simulink library "ITKLib"  (R2022b)
settings: Solver=FixedStepDiscrete  StartTime=0.0  StopTime=10.0  FixedStep=0.01  RelTol=1e-3  EnableMultiTasking=on
values from neighbouring files (symbols this model uses):
  Glb_WhlRollgRd_SC = single(0.36)    [init_Global.m]
undefined symbols (not defined in the file or in its folder): docblock, SlDemoSign, SlDemoSign_Positive_SC, TaskTime_100ms_SC, TaskTime_10ms_SC, VehRefSpd_vMaxRefSpd_C
libraries: simulink x51, $bdroot x45, ITKLib_V14 x1
(part 3 of 10)

== system ITKLib/TimeCounter ==
  Accum : Subsystem  RTWFcnName=Accum  RTWFileName=MCC_Mdl_Lib  mask(Accum){}
      mask help:
      | The main purpose of the Accum module is to achieve the accumulation of single floating-point data. Usually, when a large floating-point data is added to a small floating-point data, the data precision will be lost and the accumulation will not be possible. At this time, the small floating-point data can be accumulated separately into a large floating-point data (IncLim), and then added with another large floating-point data;
      | Input signals:
      | In : single data type, small floating-point data, for example 0.01 0.001 0.0001;
      | IncLim: single data type, the upper limiter of increasing step, for example 0.1 1 10;
      | Rst: single data type, reset flag, when Rst is true, the out is 0;
      | IV: single data type, intial value;
      | Output signals:
      | Out: single data type;
      |
      | For example, In = 0.01, IncLim = 1,
      | if without this module, when the maximum accumulation value is 100000;
      | if with this module, the maximum accumulation value is 9999999999;
      |
      | Simulink Custom Model Library, created by MCC and YZK.
      settings: MinAlgLoopOccurrences=on  RTWFcnNameOpts=User specified  RTWFileNameOpts=User specified
      mask Display:
      | color('red')
      | % plot(0.15+0.05*[0 1 1 3 3 5 5 7 7 9 9 11 11 13 13 15 15 16],0.15+0.1*[0 0 2 2 4 4 0 0 2 2 4 4 6 6 8 8 0 0] )
      | % color('blue')
      | % text(0.25,0.15,'IV')
      | color('green');
      | image('AccumImage.jpg', [0.15, 0.1, 0.75, 0.8]);
      | text(1,0,'ITK','horizontalAlignment','right','verticalAlignment','bottom');
  CountR : Subsystem  RTWFcnName=CountR  RTWFileName=BoschITK_Mdl_Lib  mask(CountR){MAX=uint16(400)}
      mask prompts: MAX "Maximum value of counter"
      mask help:
      | Increments and outputs the counter every calling (step) by value 1 when enabled and set saturation flag to TRUE when counter reaches limit.
      |
      | Reset by external request.
      |
      | Simulink Custom Model Library, created by MCC.
      settings: RTWFcnNameOpts=User specified  RTWFileNameOpts=User specified
      settings: AttributesFormatString=|
      | CountR
      | Cnt_Max=%<MAX>
      mask Display:
      | color('red')
      | plot(0.15+0.05*[0 1 1 2 2 3 3 4 4 5 5 6 6 7 7 8 8 9 9 10 10 11 11 12 12 13 13 14],0.15+0.1*[0 0 1 1 2 2 3 3 4 4 0 0 1 1 2 2 3 3 4 4 5 5 6 6 7 7 0 0] )
      | color('green');
      | text(1,0,'ITK','horizontalAlignment','right','verticalAlignment','bottom');
  CountRIV : Subsystem  RTWFcnName=CountR_IV  RTWFileName=BoschITK_Mdl_Lib  mask(CountRIV){MAX=uint16(400)}
      mask prompts: MAX "Maximum value of counter"
      mask help:
      | Increments and outputs the counter by value 1 which starts from an initial value every calling (step) when enabled and set saturation flag to TRUE when counter reaches limit.
      |
      | Reset by external request.
      |
      | Simulink Custom Model Library, created by MCC.
      settings: RTWFcnNameOpts=User specified  RTWFileNameOpts=User specified
      settings: AttributesFormatString=|
      | CountRIV
      | Cnt_Max=%<MAX>
      mask Display:
      | color('red')
      | plot(0.15+0.05*[0 1 1 2 2 3 3 4 4 5 5 6 6 7 7 8 8 9 9 10 10 11 11 12 12 13 13 14],0.15+0.1*[0 0 1 1 2 2 3 3 4 4 0 0 1 1 2 2 3 3 4 4 5 5 6 6 7 7 0 0] )
      | color('blue')
      | text(0.25,0.15,'IV')
      | color('green');
      | text(1,0,'ITK','horizontalAlignment','right','verticalAlignment','bottom');
  CounterRStep : Subsystem  RTWFcnName=CounterR_Step  RTWFileName=BoschITK_Mdl_Lib  mask(CounterRStep){Cnt_Max=uint16(400)}
      mask prompts: Cnt_Max "Maximum value of counter"
      mask help:
      | Increments and outputs the counter every calling (step) by value "Inc" when enabled and set saturation flag to TRUE when counter reaches limit.
      |
      | Reset by external request.
      |
      | Simulink Custom Model Library, created by MCC.
      mask init:
      | if Cnt_Max > 65535;
      |     helpdlg('Cnt_Max cannot be greater than 4294967295 !','ERROR1');
      | end
      | Cnt_Max = min(Cnt_Max,65535);
      settings: RTWFcnNameOpts=User specified  RTWFileNameOpts=User specified
      settings: AttributesFormatString=|
      | CounterRStep
      | Cnt_Max=%<Cnt_Max>
      mask Display:
      | color('red')
      | plot(0,0,100,100,[12,10,8,10,10],[87,90,87,90,10],[88,90,88,90,10],[7,10,12,10,10],[90,80,80,70,70,60,60,50,50,40,40,30,30,20,20],[80,80,70,70,60,60,50,50,40,40,30,30,20,20,10])
      | color('green');
      | text(100,0,'ITK','horizontalAlignment','right','verticalAlignment','bottom');
  DebCnt : Subsystem  RTWFcnName=Debounce_OBD  RTWFileName=JaevRI_Mdl_Lib  mask(DebCnt){}
      mask help:
      | Inputs:
      |              bErr: Error signal(s)  (i.e. vector of continuous test runs), boolean signal;
      |              FailThd: counter a value (for each bErr signal), int16 signal;
      |              RcvThd: counter a value (for each bErr signal), int16 signal;
      |              IncFail: increment Fault counter, >0, int16 signal;
      |              DecRcv: decrement Recovery counter, <0, int16 signal;
      |              bEna: bErr is 0 when bEna=0, detecting whether bErr is 1 when bEna=1, boolean signal;
      |              bRst: reset flag of bErr(bErr is 0 when bRst=1), boolean signal;
      | Outputs :
      |                 bFaild: testFaild  (Bit 0)
      | So Counters are in numbers of timer ticks of TaskTime( for example, 0.01s);
      | E.g. if FailThd is 20, RecThd is -4, Increment counter is 5 and decrement counter -3 when bEna is 1and bRst is 0, the initial counter is 0,
      | then fail times are: 20*0.01/5 = 0.04 sec, recovery times are: (-4-20)*0.01/(-3) = 0.08 sec;
      |
      | Simulink Custom Model Library, created by MCC.
      settings: RTWFcnNameOpts=User specified  RTWFileNameOpts=User specified
      mask Display:
      | % color('black');
      | % plot([0.2,0.2],[0.1,0.9]);
      | % plot([0.205,0.205],[0.1,0.9]);
      | % plot([0.2,0.8],[0.8,0.8]);
      | % plot([0.2,0.8],[0.65,0.65]);
      | % plot([0.2,0.8],[0.45,0.45]);
      | % plot([0.2,0.8],[0.25,0.25]);
      | % plot([0.2,0.8],[0.1,0.1]);
      | port_label('input',1,'bErr');
      | port_label('input',2,'bRst');
      | port_label('input',3,'bEna');
      | port_label('input',4,'FailThd');
      | port_label('input',5,'RcvThd');
      | port_label('input',6,'IncFail');
      | port_label('input',7,'DecRcv');
      | port_label('output',1,'bFaild');
      | % color('cyan');
      | % plot([0.3,0.3],[0.1,0.9]);
      | % plot([0.4,0.4],[0.1,0.9]);
      | % plot([0.5,0.5],[0.1,0.9]);
      | % plot([0.6,0.6],[0.1,0.9]);
      | % plot([0.7,0.7],[0.1,0.9]);
      | % plot([0.8,0.8],[0.1,0.9]);
      | % color('orange');
      | % plot([0.2,0.3,0.3,0.6,0.6,0.8],[0.85,0.85,0.8,0.8,0.85,0.85]);
      | % plot([0.2,0.5,0.5,0.6,0.6,0.8],[0.7,0.7,0.65,0.65,0.7,0.7]);
      | % color('blue');
      | % plot([0.2,0.3,0.4,0.5,0.5,0.6,0.7,0.8],[0.45,0.55,0.35,0.35,0.45,0.45,0.6,0.6]);
      | % color('red');
      | % plot([0.2,0.7,0.7,0.8],[0.25,0.25,0.3,0.3]);
      | % color('green');
      | % plot([0.2,0.4,0.4,0.5,0.5,0.8],[0.1,0.1,0.15,0.15,0.1,0.1]);
      | color('green');
      | text(1,0,'ITK','horizontalAlignment','right','verticalAlignment','bottom');
  Debounce : Subsystem  RTWFcnName=Debounce  RTWFileName=BoschITK_Mdl_Lib  mask(Debounce){IV=0}
      mask prompts: IV "Initial output value"
      mask help:
      | This block enables debounce action of input signal "In" :
      | - if it changes from fasle to true, "Out" will be set to true after TAct time
      | - if it changes from true to false, "Out" will be set to fasle after TDeact temps
      | - The initial value is given via the parameter window
      |
      | Besides,
      | "In" -- boolean type
      | R -- Reset flag，boolean type
      | TAct -- time in s, single type
      | TDeact -- time in s, single type
      | dT -- Sample time in s, single type
      |
      | Simulink Custom Model Library, created by MCC.
      mask init:
      | %val = get_param(gcb, 'IV');
      | %set_param([gcb, '/RS Latch'], 'IV', num2str(val))
      settings: RTWFcnNameOpts=User specified  RTWFileNameOpts=User specified
      settings: AttributesFormatString=|
      | Debounce
      | Init = %<IV>
      mask Display:
      | color('red')
      | plot([0.10 0.20 0.20],[0.55 0.55 0.75])
      | plot([0.20 0.22 0.22],[0.75 0.75 0.55])
      | plot([0.22 0.24 0.24],[0.55 0.55 0.75])
      | plot([0.24 0.26 0.26],[0.75 0.75 0.55])
      | plot([0.26 0.28 0.28],[0.55 0.55 0.75])
      | plot([0.28 0.70 0.70],[0.75 0.75 0.55])
      | plot([0.70 0.72 0.72],[0.55 0.55 0.75])
      | plot([0.72 0.74 0.74],[0.75 0.75 0.55])
      | plot([0.74 0.76 0.76],[0.55 0.55 0.75])
      | plot([0.76 0.78 0.78 0.90],[0.75 0.75 0.55 0.55])
      | plot([0.10 0.28 0.28],[0.25 0.25 0.45])
      | plot([0.28 0.78 0.78 0.90],[0.45 0.45 0.25 0.25])
      | color('black')
      | plot([0.20 0.27],[0.55 0.75])
      | plot([0.20 0.27],[0.75 0.55])
      | plot([0.70 0.78],[0.55 0.75])
      | plot([0.70 0.78],[0.75 0.55])
      | color('green')
      | text(1,0,'ITK','horizontalAlignment','right','verticalAlignment','bottom')
  InDly : Stateflow chart  TreatAsAtomicUnit=on  mask(InDly){}
      mask help:
      | The module can delay the input In by DlyCnt steps before outputting it..
      | Input signals:
      |             In: input signal, single data type;
      |             DlyCnt: delay counter value, uint16 data type;
      |
      | Output signals:
      |             InDly: the input value delayed by DlyCnt steps, single data type;
      |
      | the dimension of InDlyAry is [1 DlyCnt+10].
      | For example, if DlyCnt= 10.
      | in the step from 0 to DlyCnt, InDly = In;
      | after step from 10, InDly equals the input In from DlyCnt steps earlier.
      |
      | Simulink Custom Model Library, created by MCC.
  StopWatchRE : Subsystem  Description=""  RTWFcnName=StopWatchRE  RTWFileName=BoschITK_Mdl_Lib  mask(StopWatchRE){}
      mask help:
      | The block outputs the time since the system init or the last reset.
      | Simulink Custom Model Library, created by MCC.
      settings: RTWFcnNameOpts=User specified  RTWFileNameOpts=User specified
      mask Display:
      | color('black');
      | plot(0.5+0.35*cos(0:pi/12:2*pi),0.5+0.35*sin(0:pi/12:2*pi));
      | plot([0.5,0.5],[0.85,0.75]);
      | plot([0.5,0.5],[0.15,0.25]);
      | plot([0.15,0.25],[0.5,0.5]);
      | plot([0.75,0.85],[0.5,0.5]);
      | color('red');
      | plot([0.5,0.5+0.25*cos(pi/4)],[0.5,0.5+0.25*sin(pi/4)]);
      | plot([0.5,0.5+0.15*cos(pi*3/2)],[0.5,0.5+0.15*sin(pi*3/2)]);
      | plot(0.5+0.02*cos(0:pi/12:2*pi),0.5+0.02*sin(0:pi/12:2*pi));
      | color('green');
      | text(1,0,'ITK','horizontalAlignment','right','verticalAlignment','bottom');
  TurnOnDelayVari : Subsystem  RTWFcnName=TurnOn_Delay  RTWFileName=BoschITK_Mdl_Lib  mask(TurnOnDelay){}
      mask help:
      | Turn on delay with variant delay time
      | Input signal is passed from port 'u'
      | Sample time is passed from 'dT'
      | Variant delay time is passed from 'T'
      | First Step Delay Enable is given in the parameters
      |
      | The rising edge of input signal is delayed for a given time.
      | When First Step Delay Enable is 1, the input signal will be recognized as the rising edge if it is 0 at the first step.
      |
      | Simulink Custom Model Library, created by MCC.
      settings: AttributesFormatString=TurnOnDelay
      mask Help:
      | Turn on delay with variant delay time
      | Input signal is passed from port 'u'
      | Sample time is passed from 'dT'
      | Variant delay time is passed from 'T'
      | First Step Delay Enable is given in the parameters
      | 
      | The rising edge of input signal is delayed for a given time.
      | When First Step Delay Enable is 1, the input signal will be recognized as the rising edge if it is 0 at the first step.
      mask Display:
      | color('blue')
      | disp('\fontsize{16}T', 'texmode', 'on')
      | color('red')
      | plot([0.2 0.6 0.6 0.8], [0.2 0.2 0.8 0.8])
      | plot([0.4 0.4],[0.25 0.35])
      | plot([0.4 0.4],[0.45 0.55])
      | plot([0.4 0.4],[0.65 0.75])
      | plot([0.425 0.475],[0.8 0.8])
      | plot([0.525 0.575],[0.8 0.8])
      | color('black')
      | port_label('input', 1, 'In', 'texmode', 'on')
      | port_label('input', 2, 'dT', 'texmode', 'on')
      | port_label('input', 3, 'T', 'texmode', 'on')
      | port_label('output', 1, 'Out', 'texmode', 'on')
      | color('green');
      | text(1,0,'ITK','horizontalAlignment','right','verticalAlignment','bottom');
  Turn_Off_Delay_Vari : Subsystem  RTWFcnName=TurnOff_Delay  RTWFileName=BoschITK_Mdl_Lib  mask(TurnOffDelay){}
      mask help:
      | Turn off delay with variant delay time
      | Input signal is passed from port 'u'
      | Sample time is passed from 'dT'
      | Variant delay time is passed from 'T'.
      | First Step Delay is given in the parameters
      |
      | The falling edge of input signal is delayed for a given time.
      | hen First Step Delay Enable is 1, the input signal will be recognized as the falling edge if it is 0 at the first step.
      |
      | Simulink Custom Model Library, created by MCC.
      settings: AttributesFormatString=TurnOffDelay  RTWFcnNameOpts=User specified  RTWFileNameOpts=User specified
      mask Help:
      | Turn off delay with variant delay time
      | Input signal is passed from port 'u'
      | Sample time is passed from 'dT'
      | Variant delay time is passed from 'T'
      | First Step Delay Enable is given in the parameters
      | 
      | The falling edge of input signal is delayed for a given time.
      | When First Step Delay Enable is 1, the input signal will be recognized as the falling edge if it is 0 at the first step.
      mask Display:
      | color('blue')
      | disp('\fontsize{16}T', 'texmode', 'on')
      | color('red')
      | plot([0.2 0.4 0.4 0.8], [0.8 0.8 0.2 0.2])
      | plot([0.425 0.48],[0.8 0.8])
      | plot([0.55 0.6],[0.8 0.8])
      | plot([0.65 0.65],[0.8 0.7])
      | plot([0.65 0.65],[0.65 0.55])
      | plot([0.65 0.65],[0.5 0.4])
      | plot([0.65 0.65],[0.35 0.25])
      | color('black')
      | port_label('input', 1, 'In', 'texmode', 'on')
      | port_label('input', 2, 'dT', 'texmode', 'on')
      | port_label('input', 3, 'T', 'texmode', 'on')
      | port_label('output', 1, 'Out', 'texmode', 'on')
      | color('green');
      | text(1,0,'ITK','horizontalAlignment','right','verticalAlignment','bottom');
  Variable Integer Delay1 : Delay  DelayLengthSource=Input port  DelayLengthUpperLimit=200  UseCircularBuffer=on
      settings: InputPortMap=u0,p1
  trig_TaskTime_A : Stateflow chart  Description=trig_TaskTime_A  RTWFcnName=trig_TaskTime_A  RTWFileName=BoschITK_Mdl_Lib
      settings: AttributesFormatString=%<Description>  RTWSystemCode=Reusable function  RTWFcnNameOpts=User specified  RTWFileNameOpts=User specified
  trig_TaskTime_B : Stateflow chart  Description=trig_TaskTime_B  RTWFcnName=trig_TaskTime_B  RTWFileName=BoschITK_Mdl_Lib
      settings: AttributesFormatString=%<Description>  RTWSystemCode=Reusable function  RTWFcnNameOpts=User specified  RTWFileNameOpts=User specified

== system ITKLib/BasicOperators/AbsITK ==
  In1 : Inport
  Greater : RelationalOperator  Operator=>  OutDataTypeStr=boolean
  Product : Product  InputSameDT=on  SaturateOnIntegerOverflow=on
  Switch : Switch  Criteria=u2 ~= 0  SaturateOnIntegerOverflow=off  InputSameDT=off
      settings: AttributesFormatString=Criteria : %<Criteria>
  single : Constant  Value=0  OutDataTypeStr=single  SampleTime=-1
      settings: AttributesFormatString=%<OutDataTypeStr>
  single1 : Constant  Value=-1  OutDataTypeStr=single  SampleTime=-1
      settings: AttributesFormatString=%<OutDataTypeStr>
  Out1 : Outport  VectorParamsAs1DForOutWhenUnconnected=off
  wires:
  In1/1 -> Greater/1, Product/1, Switch/1
  Greater/1 -> Switch/2
  Switch/1 -> Out1/1
  single/1 -> Greater/2
  single1/1 -> Product/2
  Product/1 -> Switch/3

== system ITKLib/BasicOperators/AcosDeg ==
  u : Inport
  1-D Lookup Table1 : Lookup_n-D  NumberOfTableDimensions=1  BreakpointsForDimension1=[0,0.05,0.1,0.15,0.2,0.25,0.3,0.35,0.4,0.45,0.5,0.55,0.6,0.65,0.7,0.75,0.8,0.85,0.9,0.95,1]  BreakpointsForDimension1DataTypeStr=single  Table=[90,87.1340160174012,84.2608295227332,81.3730734413214,78.4630409671845,75.5224878140701,72.5423968762779,69.5126848852773,66.4218215217982,63.2563160495970,60.0000000000000,56.6329870307682,53.1301023541560,49.4583981264955,45.5729959991943,41.4096221092709,36.8698976458440,31.7883306170516,25.8419327631671,18.1948723387668,0]  TableDataTypeStr=single  IntermediateResultsDataTypeStr=single  ExtrapMethod=Clip  UseLastTableValue=on  InternalRulePriority=Speed  OutDataTypeStr=single  RndMeth=Simplest  FractionDataTypeStr=single
      settings: AttributesFormatString=|
      | input = %<BreakpointsForDimension1>
      | output = %<Table>
      | extrapolation-use end values: %<UseLastTableValue>
  AbsITK : $bdroot/BasicOperators/AbsITK
  GreaterOrEqual3 : RelationalOperator  OutDataTypeStr=boolean
  Subtract : Sum  Inputs=+-  InputSameDT=on  SaturateOnIntegerOverflow=on
  Switch1 : Switch  Criteria=u2 ~= 0  SaturateOnIntegerOverflow=off  InputSameDT=off
      settings: AttributesFormatString=Criteria : %<Criteria>
  single1 : Constant  Value=0  OutDataTypeStr=single
      settings: AttributesFormatString=%<OutDataTypeStr>
  single2 : Constant  Value=180  OutDataTypeStr=single
      settings: AttributesFormatString=%<OutDataTypeStr>
  deg : Outport
  wires:
  u/1 -> AbsITK/1, GreaterOrEqual3/1
  Switch1/1 -> deg/1
  Subtract/1 -> Switch1/3
  single2/1 -> Subtract/1
  1-D Lookup Table1/1 -> Subtract/2, Switch1/1
  GreaterOrEqual3/1 -> Switch1/2
  single1/1 -> GreaterOrEqual3/2
  AbsITK/1 -> 1-D Lookup Table1/1

== system ITKLib/BasicOperators/AsinDeg ==
  u : Inport
  1-D Lookup Table1 : Lookup_n-D  NumberOfTableDimensions=1  BreakpointsForDimension1=[0,0.05,0.1,0.15,0.2,0.25,0.3,0.35,0.4,0.45,0.5,0.55,0.6,0.65,0.7,0.75,0.8,0.85,0.9,0.95,1]  BreakpointsForDimension1DataTypeStr=single  Table=[0,2.86598398259886,5.73917047726679,8.62692655867864,11.5369590328155,14.4775121859299,17.4576031237221,20.4873151147227,23.5781784782018,26.7436839504030,30.0000000000000,33.3670129692318,36.8698976458440,40.5416018735045,44.4270040008057,48.5903778907291,53.1301023541560,58.2116693829484,64.1580672368329,71.8051276612332,90]  TableDataTypeStr=single  IntermediateResultsDataTypeStr=single  ExtrapMethod=Clip  UseLastTableValue=on  InternalRulePriority=Speed  OutDataTypeStr=single  RndMeth=Simplest  FractionDataTypeStr=single
      settings: AttributesFormatString=|
      | input = %<BreakpointsForDimension1>
      | output = %<Table>
      | extrapolation-use end values: %<UseLastTableValue>
  AbsITK : $bdroot/BasicOperators/AbsITK
  GreaterOrEqual3 : RelationalOperator  OutDataTypeStr=boolean
  Product : Product  InputSameDT=on  RndMeth=Zero  SaturateOnIntegerOverflow=on
  Switch1 : Switch  Criteria=u2 ~= 0  SaturateOnIntegerOverflow=off  InputSameDT=off
      settings: AttributesFormatString=Criteria : %<Criteria>
  single1 : Constant  Value=0  OutDataTypeStr=single
      settings: AttributesFormatString=%<OutDataTypeStr>
  single2 : Constant  Value=-1  OutDataTypeStr=single
      settings: AttributesFormatString=%<OutDataTypeStr>
  deg : Outport
  wires:
  single1/1 -> GreaterOrEqual3/2
  GreaterOrEqual3/1 -> Switch1/2
  1-D Lookup Table1/1 -> Switch1/1, Product/1
  single2/1 -> Product/2
  Product/1 -> Switch1/3
  Switch1/1 -> deg/1
  u/1 -> AbsITK/1, GreaterOrEqual3/1
  AbsITK/1 -> 1-D Lookup Table1/1

== system ITKLib/BasicOperators/Atan2Deg ==
  y : Inport
  x : Inport  Port=2
  1-D Lookup Table3 : Lookup_n-D  NumberOfTableDimensions=1  BreakpointsForDimension1=[0,0.00153414561609111,0.00306829845373796,0.00460246573463227,0.00613665468073772,0.00767087251442592,0.00920512645861245,0.0107394237368928,0.0122737715736787,0.0138081771943337,0.0153426478253099,0.0168771906942835,0.0184118130302918,0.0199465220638685,0.0214813250271809,0.0230162291541658,0.0245512416806661,0.0260863698445676,0.0276216208859351,0.0291570020471495,0.0306925205730446,0.0322281837110438,0.0337639987112974,0.0352999728268193,0.0368361133136247,0.0383724274308672,0.0399089224409762,0.0414456056097949,0.0429824842067175,0.0445195655048274,0.0460568567810355,0.0475943653162178,0.0491320983953542,0.0506700633076669,0.0522082673467589,0.0537467178107533,0.0552854220024318,0.0568243872293744,0.0583636208040985,0.0599031300441989,0.0614429222724871,0.0629830048171318,0.0645233850117991,0.0660640701957925,0.0676050677141943,0.0691463849180061,0.0706880291642902,0.0722300078163106,0.0737723282436753,0.0753149978224779,0.0768580239354395,0.0784014139720518,0.0799451753287194,0.0814893154089027,0.0830338416232617,0.0845787613897992,0.0861240821340046,0.0876698112889985,0.089215956295677,0.0907625246028563,0.0923095236674182,0.0938569609544554,0.0954048439374171,0.0969531800982557,0.0985019769275727,0.100051241924766,0.101600982598176,0.103151206465235,0.104701921052615,0.106253133896373,0.107804852542103,0.109357084545084,0.11090983747043,0.112463118893239,0.114016936398742,0.115571297582457,0.117126210050339,0.11868168141893,0.120237719315512,0.12179433137826,0.123351525256394,0.124909308610333,0.126467689111848,0.128026674444216,0.129586272302379,0.131146490393091,0.132707336435082,0.134268818159209,0.135830943308615,0.137393719638886,0.138957154918206,0.140521256927521,0.142086033460691,0.143651492324657,0.145217641339592,0.146784488339068,0.148352041170216,0.149920307693886,0.151489295784808,0.153059013331758,0.15462946823772,0.156200668420048,0.157772621810633,0.159345336356066,0.160918820017808,0.162493080772349,0.164068126611382,0.165643965541967,0.167220605586699,0.168798054783879,0.170376321187682,0.171955412868328,0.173535337912253,0.175116104422279,0.176697720517789,0.178280194334898,0.179863534026628,0.181447747763079,0.183032843731611,0.184618830137013,0.186205715201682,0.187793507165804,0.189382214287526,0.19097184484314,0.192562407127258,0.194153909452998,0.195746360152162,0.197339767575415,0.198934140092477,0.200529486092297,0.202125813983243,0.203723132193287,0.205321449170188,0.206920773381683,0.208521113315675,0.210122477480416,0.211724874404705,0.213328312638072,0.214932800750974,0.216538347334983,0.218144961002985,0.219752650389369,0.221361424150224,0.222971290963538,0.22458225952939,0.226194338570153,0.227807536830688,0.229421863078552,0.231037326104188,0.232653934721138,0.234271697766238,0.235890624099828,0.237510722605954,0.239132002192573,0.240754471791765,0.242378140359935,0.244003016878031,0.245629110351746,0.247256429811733,0.24888498431382,0.250514782939222,0.252145834794754,0.253778149013052,0.255411734752785,0.257046601198878,0.258682757562729,0.260320213082433,0.261958977022998,0.263599058676576,0.265240467362683,0.266883212428424,0.268527303248726,0.270172749226557,0.271819559793166,0.273467744408305,0.275117312560467,0.276768273767119,0.278420637574933,0.280074413560027,0.281729611328199,0.283386240515168,0.285044310786815,0.286703831839422,0.288364813399917,0.290027265226121,0.291691197106988,0.293356618862858,0.295023540345704,0.29669197143938,0.298361922059879,0.300033402155581,0.30170642170751,0.303380990729589,0.305057119268901,0.306734817405947,0.308414095254907,0.310094962963901,0.311777430715259,0.313461508725781,0.315147207247009,0.316834536565492,0.318523507003062,0.320214128917103,0.321906412700828,0.323600368783554,0.325296007630978,0.32699333974546,0.328692375666303,0.330393125970036,0.332095601270698,0.333799812220128,0.33550576950825,0.337213483863366,0.338922966052449,0.340634226881433,0.342347277195516,0.344062127879451,0.345778789857851,0.347497274095491 ...(+13906 chars)]  BreakpointsForDimension1DataTypeStr=single  Table=[0,0.0879,0.1758,0.2637,0.3516,0.4395,0.5274,0.6153,0.7032,0.7911,0.879,0.9669,1.0548,1.1427,1.2306,1.3185,1.4064,1.4943,1.5822,1.6701,1.758,1.8459,1.9338,2.0217,2.1096,2.1975,2.2854,2.3733,2.4612,2.5491,2.637,2.7249,2.8128,2.9007,2.9886,3.0765,3.1644,3.2523,3.3402,3.4281,3.516,3.6039,3.6918,3.7797,3.8676,3.9555,4.0434,4.1313,4.2192,4.3071,4.395,4.4829,4.5708,4.6587,4.7466,4.8345,4.9224,5.0103,5.0982,5.1861,5.274,5.3619,5.4498,5.5377,5.6256,5.7135,5.8014,5.8893,5.9772,6.0651,6.153,6.2409,6.3288,6.4167,6.5046,6.5925,6.6804,6.7683,6.8562,6.9441,7.032,7.1199,7.2078,7.2957,7.3836,7.4715,7.5594,7.6473,7.7352,7.8231,7.911,7.9989,8.0868,8.1747,8.2626,8.3505,8.4384,8.5263,8.6142,8.7021,8.79,8.8779,8.9658,9.0537,9.1416,9.2295,9.3174,9.4053,9.4932,9.5811,9.669,9.7569,9.8448,9.9327,10.0206,10.1085,10.1964,10.2843,10.3722,10.4601,10.548,10.6359,10.7238,10.8117,10.8996,10.9875,11.0754,11.1633,11.2512,11.3391,11.427,11.5149,11.6028,11.6907,11.7786,11.8665,11.9544,12.0423,12.1302,12.2181,12.306,12.3939,12.4818,12.5697,12.6576,12.7455,12.8334,12.9213,13.0092,13.0971,13.185,13.2729,13.3608,13.4487,13.5366,13.6245,13.7124,13.8003,13.8882,13.9761,14.064,14.1519,14.2398,14.3277,14.4156,14.5035,14.5914,14.6793,14.7672,14.8551,14.943,15.0309,15.1188,15.2067,15.2946,15.3825,15.4704,15.5583,15.6462,15.7341,15.822,15.9099,15.9978,16.0857,16.1736,16.2615,16.3494,16.4373,16.5252,16.6131,16.701,16.7889,16.8768,16.9647,17.0526,17.1405,17.2284,17.3163,17.4042,17.4921,17.58,17.6679,17.7558,17.8437,17.9316,18.0195,18.1074,18.1953,18.2832,18.3711,18.459,18.5469,18.6348,18.7227,18.8106,18.8985,18.9864,19.0743,19.1622,19.2501,19.338,19.4259,19.5138,19.6017,19.6896,19.7775,19.8654,19.9533,20.0412,20.1291,20.217,20.3049,20.3928,20.4807,20.5686,20.6565,20.7444,20.8323,20.9202,21.0081,21.096,21.1839,21.2718,21.3597,21.4476,21.5355,21.6234,21.7113,21.7992,21.8871,21.975,22.0629,22.1508,22.2387,22.3266,22.4145,22.5024,22.5903,22.6782,22.7661,22.854,22.9419,23.0298,23.1177,23.2056,23.2935,23.3814,23.4693,23.5572,23.6451,23.733,23.8209,23.9088,23.9967,24.0846,24.1725,24.2604,24.3483,24.4362,24.5241,24.612,24.6999,24.7878,24.8757,24.9636,25.0515,25.1394,25.2273,25.3152,25.4031,25.491,25.5789,25.6668,25.7547,25.8426,25.9305,26.0184,26.1063,26.1942,26.2821,26.37,26.4579,26.5458,26.6337,26.7216,26.8095,26.8974,26.9853,27.0732,27.1611,27.249,27.3369,27.4248,27.5127,27.6006,27.6885,27.7764,27.8643,27.9522,28.0401,28.128,28.2159,28.3038,28.3917,28.4796,28.5675,28.6554,28.7433,28.8312,28.9191,29.007,29.0949,29.1828,29.2707,29.3586,29.4465,29.5344,29.6223,29.7102,29.7981,29.886,29.9739,30.0618,30.1497,30.2376,30.3255,30.4134,30.5013,30.5892,30.6771,30.765,30.8529,30.9408,31.0287,31.1166,31.2045,31.2924,31.3803,31.4682,31.5561,31.644,31.7319,31.8198,31.9077,31.9956,32.0835,32.1714,32.2593,32.3472,32.4351,32.523,32.6109,32.6988,32.7867,32.8746,32.9625,33.0504,33.1383,33.2262,33.3141,33.402,33.4899,33.5778,33.6657,33.7536,33.8415,33.9294,34.0173,34.1052,34.1931,34.281,34.3689,34.4568,34.5447,34.6326,34.7205,34.8084,34.8963,34.9842,35.0721,35.16,35.2479,35.3358,35.4237,35.5116,35.5995,35.6874,35.7753,35.8632,35.9511,36.039,36.1269,36.2148,36.3027,36.3906,36.4785,36.5664,36.6543,36.7422,36.8301,36.918,37.0059,37.0938,37.1817,37.2696,37.3575,37.4454,37.5333,37.6212,37.7091,37.797,37.8849,37.9728,38.0607,38.1486,38.2365,38.3244,38.4123,38.5002,38.5881,38.676,38.7639,38.8518,38.9397,39.0276,39.1155,39.2034,39.2913,39.3792,39.4671,39.555,39.6429,39.7308,39.8187,39.9066,39.9945,40.0824,40.1703,40.2582,40.3461,40.434,40.5219,40.6098,40.6977,40.7856,40.8735,40.9614,41.0493,41.1372,41.2251,41.313,41.4009,41.4888,41.5767,41.6646,41.7525,41.8404,41.9283,42.0162,42.1041,42.192,42.2799,42.3678,42.4557,42.5436,42.6315,42.7194,42.8073,42.8952,42.9831,43.071,43.1589,43.2468,43.3347,43.4226,43.5105,43.5984,43.6863,43.7742,43.8621,43.95,44.0379,44.1258,44.2137,44.3016,44.3895,44.4774,44.5653,44.6532,44.7411,44.829,44.9169,45.0048,45.0927,45.1806,45.2685,45.3564,45.4443,45.5322,45.6201,45.708 ...(+3974 chars)]  TableDataTypeStr=single  IntermediateResultsDataTypeStr=single  ExtrapMethod=Clip  UseLastTableValue=on  InternalRulePriority=Speed  OutDataTypeStr=single  RndMeth=Simplest  FractionDataTypeStr=single
      settings: AttributesFormatString=|
      | input = %<BreakpointsForDimension1>
      | output = %<Table>
      | extrapolation-use end values: %<UseLastTableValue>
  AND{,1..3} (4 alike) : Logic  OutDataTypeStr=boolean
  AbsITK : $bdroot/BasicOperators/AbsITK
  Add : Sum  InputSameDT=on  SaturateOnIntegerOverflow=on
  GreaterOrEqual{1,6..8} (4 alike) : RelationalOperator  Operator=<  OutDataTypeStr=boolean
  GreaterOrEqual{3..5,9} (4 alike) : RelationalOperator  OutDataTypeStr=boolean
  Opposite : $bdroot/BasicOperators/Opposite
  Safe_Divide : $bdroot/BasicOperators/Safe_Divide
  Subtract : Sum  Inputs=+-  InputSameDT=on  SaturateOnIntegerOverflow=on
  Switch{1,4..6} (4 alike) : Switch  Criteria=u2 ~= 0  SaturateOnIntegerOverflow=off  InputSameDT=off
      settings: AttributesFormatString=Criteria : %<Criteria>
  single : Constant  Value=0.001  OutDataTypeStr=single
      settings: AttributesFormatString=%<OutDataTypeStr>
  single{1..3,6,8,10,12..13} (8 alike) : Constant  Value=0  OutDataTypeStr=single
      settings: AttributesFormatString=%<OutDataTypeStr>
  single11 : Constant  Value=-180  OutDataTypeStr=single
      settings: AttributesFormatString=%<OutDataTypeStr>
  single9 : Constant  Value=180  OutDataTypeStr=single
      settings: AttributesFormatString=%<OutDataTypeStr>
  deg : Outport
  wires:
  Safe_Divide/1 -> AbsITK/1
  Switch1/1 -> deg/1
  Switch4/1 -> Switch1/3
  1-D Lookup Table3/1 -> [AgAbs], Switch1/1
  y/1 -> Safe_Divide/1, [y]
  x/1 -> [x], Safe_Divide/2
  single/1 -> Safe_Divide/3
  single6/1 -> GreaterOrEqual4/2
  [y] -> GreaterOrEqual4/1
  single8/1 -> GreaterOrEqual5/2
  [x] -> GreaterOrEqual5/1
  GreaterOrEqual4/1 -> AND/1
  GreaterOrEqual5/1 -> AND/2
  AND/1 -> Switch1/2  "FirstQuadrant"
  GreaterOrEqual6/1 -> AND1/2
  GreaterOrEqual3/1 -> AND1/1
  [x] -> GreaterOrEqual6/1
  single2/1 -> GreaterOrEqual6/2
  [y] -> GreaterOrEqual3/1
  single1/1 -> GreaterOrEqual3/2
  AND1/1 -> Switch4/2  "SecondQuadrant"
  single9/1 -> Subtract/1
  [AgAbs] -> Subtract/2
  Subtract/1 -> Switch4/1
  single3/1 -> GreaterOrEqual1/2
  [y] -> GreaterOrEqual1/1
  single10/1 -> GreaterOrEqual7/2
  [x] -> GreaterOrEqual7/1
  GreaterOrEqual1/1 -> AND2/1
  GreaterOrEqual7/1 -> AND2/2
  AND2/1 -> Switch5/2  "ThirdQuadrant"
  Switch5/1 -> Switch4/3
  single11/1 -> Add/1
  Add/1 -> Switch5/1
  [AgAbs] -> Add/2
  GreaterOrEqual9/1 -> AND3/2
  GreaterOrEqual8/1 -> AND3/1
  [x] -> GreaterOrEqual9/1
  single12/1 -> GreaterOrEqual9/2
  [y] -> GreaterOrEqual8/1
  single13/1 -> GreaterOrEqual8/2
  AND3/1 -> Switch6/2  "FourthQuadrant"
  Switch6/1 -> Switch5/3
  [AgAbs] -> Opposite/1
  [AgAbs] -> Switch6/3
  Opposite/1 -> Switch6/1
  AbsITK/1 -> 1-D Lookup Table3/1
